simulink model "gm_parallel_phase_voltages_per_switching_state_6"  (R2022a)
settings: Solver=FixedStepDiscrete  StartTime=0.0  StopTime=10.0  RelTol=1e-3
undefined symbols (not defined in the file or in its folder): f_c, u_dc
libraries: hdlmdlgenlib x20
(part 1 of 5)
settings Model: Creator=Andre Merx  LastModifiedBy=Andre Merx
settings SolverCC: AlgebraicLoopSolver=TrustRegion
settings DataIOCC: LimitDataPoints=on  SaveOutput=off  SaveTime=off
settings OptimizationCC: BlockReduction=off  ConditionallyExecuteInputs=off  DefaultParameterBehavior=Inlined  LifeSpan=inf
settings DebuggingCC: AlgebraicLoopMsg=error  InheritedTsInSrcMsg=none  SingleTaskRateTransMsg=error  UnconnectedInputMsg=warning  UnconnectedOutputMsg=warning  UnconnectedLineMsg=warning  AllowSymbolicDim=off  StrictBusMsg=ErrorOnBusTreatedAsVector  SFUnexpectedBacktrackingDiag=warning  SFNoUnconditionalDefaultTransitionDiag=warning  SFExecutionAtInitializationDiag=none  SFMachineParentedDataDiag=warning  ArithmeticOperatorsInVariantConditions=warning
settings HardwareCC: ProdBitPerPointer=32  ProdBitPerSizeT=32  ProdBitPerPtrDiffT=32  ProdLargestAtomicFloat=None  ProdIntDivRoundTo=Undefined  ProdEndianess=Unspecified  ProdWordSize=32  ProdHWDeviceType=ASIC/FPGA->ASIC/FPGA  ProdEqTarget=off
settings SFSimCC: SimUseLocalCustomCode=off  CustomCodeUndefinedFunction=UseInterfaceOnly
settings RTWCC: RTWUseLocalCustomCode=off
settings CodeAppCC: StateflowObjectComments=on
settings GRTTargetCC: TargetLangStandard=C89/C90 (ANSI)
settings ConfigComp: CovScope=ReferencedModels  CovMetricSettings=dw  CovSaveCumulativeToWorkspaceVar=on  CovSaveSingleToWorkspaceVar=on  CovExternalEMLEnable=off  CovSFcnEnable=off

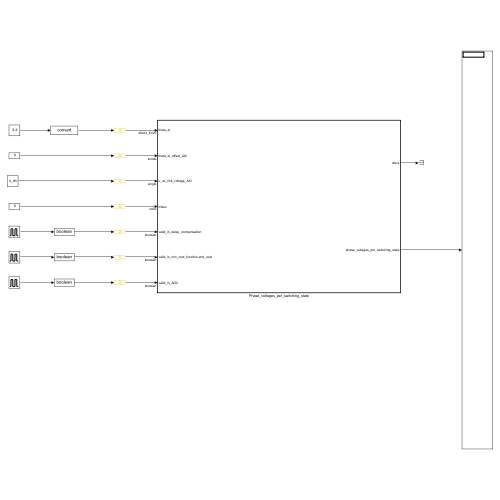
[thumbnail: Simulink's stored preview of the top-level diagram]
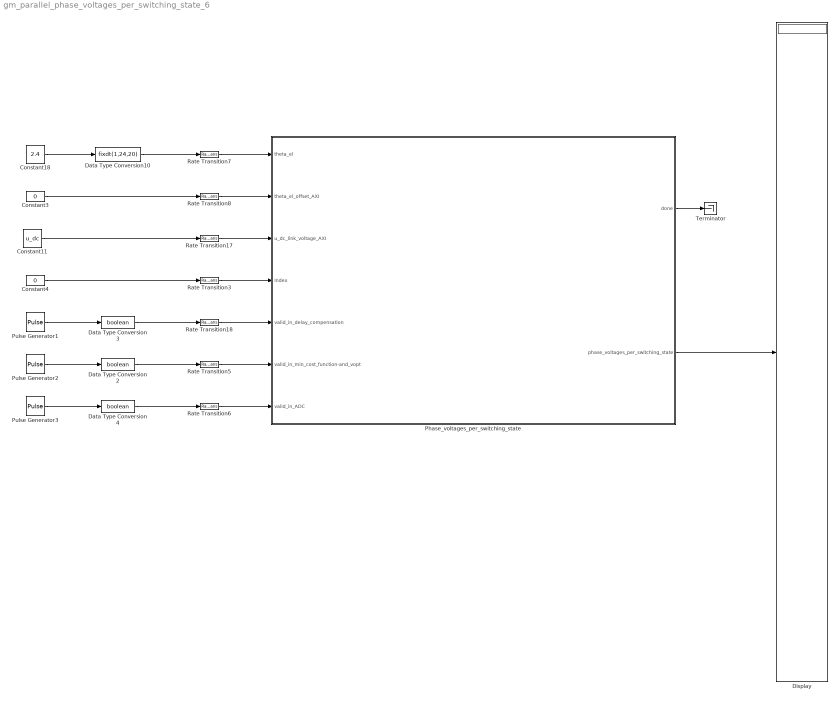
== system gm_parallel_phase_voltages_per_switching_state_6 ==
  Constant11 : Constant  Value=u_dc  OutDataTypeStr=single  SampleTime=-1
  Constant18 : Constant  Value=2.4
  Constant3 : Constant  Value=0  OutDataTypeStr=single  SampleTime=-1
  Constant4 : Constant  Value=0  OutDataTypeStr=int32  SampleTime=-1
  Data Type Conversion10 : DataTypeConversion  OutDataTypeStr=fixdt(1,24,20)  SaturateOnIntegerOverflow=off  RndMeth=Floor
  Data Type Conversion2 : DataTypeConversion  OutDataTypeStr=boolean  SaturateOnIntegerOverflow=off  RndMeth=Floor
  Data Type Conversion3 : DataTypeConversion  OutDataTypeStr=boolean  SaturateOnIntegerOverflow=off  RndMeth=Floor
  Data Type Conversion4 : DataTypeConversion  OutDataTypeStr=boolean  SaturateOnIntegerOverflow=off  RndMeth=Floor
  Display : Display
  Phase_voltages_per_switching_state : Subsystem  TreatAsAtomicUnit=on
  Pulse Generator1 : DiscretePulseGenerator  PulseType=Time based  Period=1/f_c
  Pulse Generator2 : DiscretePulseGenerator  PulseType=Time based  Period=1/f_c
  Pulse Generator3 : DiscretePulseGenerator  PulseType=Time based  Period=1/f_c
  Rate Transition{3,5..8,17..18} (7 alike) : RateTransition  OutPortSampleTime=Rt
  Terminator : Terminator
  wires:
  Phase_voltages_per_switching_state/2(phase_voltages_per_switching_state) -> Display/1
  Phase_voltages_per_switching_state/1(done) -> Terminator/1
  Data Type Conversion10/1 -> Rate Transition7/1
  Constant11/1 -> Rate Transition17/1
  Constant3/1 -> Rate Transition8/1
  Rate Transition17/1 -> Phase_voltages_per_switching_state/3(u_dc_link_voltage_AXI)
  Constant4/1 -> Rate Transition3/1
  Rate Transition7/1 -> Phase_voltages_per_switching_state/1(theta_el)
  Pulse Generator1/1 -> Data Type Conversion3/1
  Rate Transition8/1 -> Phase_voltages_per_switching_state/2(theta_el_offset_AXI)
  Constant18/1 -> Data Type Conversion10/1
  Rate Transition18/1 -> Phase_voltages_per_switching_state/5(valid_in_delay_compensation)
  Rate Transition3/1 -> Phase_voltages_per_switching_state/4(Index)
  Pulse Generator2/1 -> Data Type Conversion2/1
  Pulse Generator3/1 -> Data Type Conversion4/1
  Data Type Conversion4/1 -> Rate Transition6/1
  Rate Transition6/1 -> Phase_voltages_per_switching_state/7(valid_in_ADC)
  Rate Transition5/1 -> Phase_voltages_per_switching_state/6(valid_in_min_cost_function-and_vopt)
  Data Type Conversion3/1 -> Rate Transition18/1
  Data Type Conversion2/1 -> Rate Transition5/1

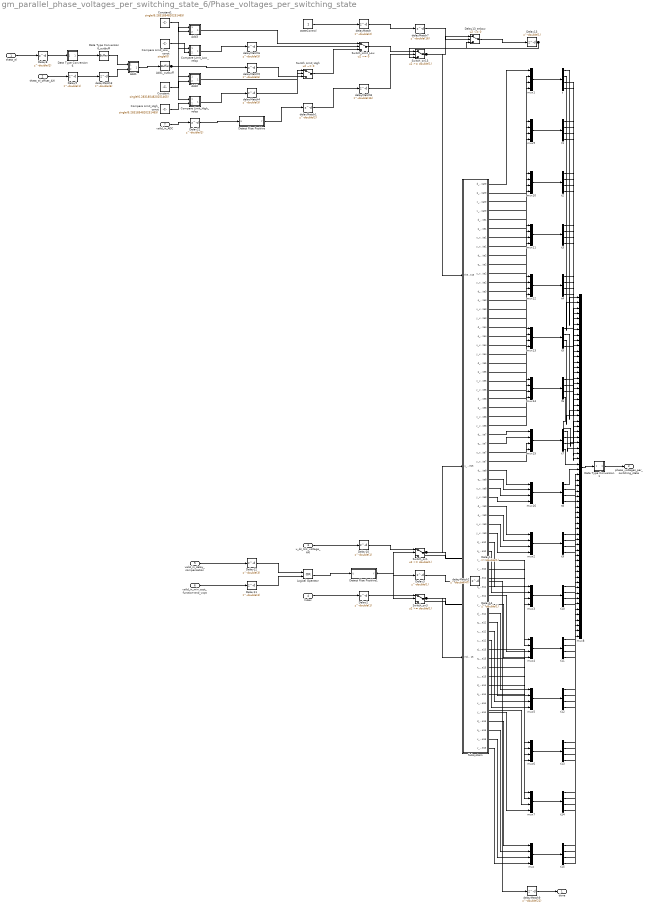
== system gm_parallel_phase_voltages_per_switching_state_6/Phase_voltages_per_switching_state ==
  theta_el : Inport  OutDataTypeStr=fixdt(1, 24, 20)  PortDimensions=1  SampleTime=1e-08
  theta_el_offset_AXI : Inport  Port=2  OutDataTypeStr=single  PortDimensions=1  SampleTime=1e-08
  u_dc_link_voltage_AXI : Inport  Port=3  OutDataTypeStr=single  PortDimensions=1  SampleTime=1e-08
  Index : Inport  Port=4  OutDataTypeStr=int32  PortDimensions=1  SampleTime=1e-08
  valid_in_delay_compensation : Inport  Port=5  OutDataTypeStr=boolean  PortDimensions=1  SampleTime=1e-08
  valid_in_min_cost_function-and_vopt : Inport  Port=6  OutDataTypeStr=boolean  PortDimensions=1  SampleTime=1e-08
  valid_in_ADC : Inport  Port=7  OutDataTypeStr=boolean  PortDimensions=1  SampleTime=1e-08
  Add1 : Subsystem
      mask Display: disp('NFP\nadd');
  Add1_outbuff : hdlmdlgenlib/Buffer
      settings: SourceProductBaseCode=SL
  Add2 : Subsystem
      mask Display: disp('NFP\nadd');
  Add3 : Subsystem
      mask Display: disp('NFP\nadd');
  Compare Limit_High_const : Constant  Value=single(6.2831854820251465)  OutDataTypeStr=single  SampleTime=1e-08
  Compare Limit_High_relop : Subsystem
      mask Display: disp('NFP\nrelop');
  Compare Limit_Low_const : Constant  Value=single(0)  OutDataTypeStr=single  SampleTime=1e-08
  Compare Limit_Low_relop : Subsystem
      mask Display: disp('NFP\nrelop');
  Constant : Constant  Value=single(6.2831854820251465)  OutDataTypeStr=single  SampleTime=1e-08
  Constant1 : Constant  Value=single(6.2831854820251465)  OutDataTypeStr=single  SampleTime=1e-08
  Data Type Conversion1 : Subsystem
      mask Display: disp('NFP\nconv');
  Data Type Conversion6 : Subsystem
      mask Display: disp('NFP\nconv');
  Data Type Conversion6_outbuff : hdlmdlgenlib/Buffer
      settings: SourceProductBaseCode=SL
  Delay{1..3,8..10,13..14,21} (9 alike) : Delay  DelayLength=double(1)  InitialCondition=0  SampleTime=1e-08
  Delay11 : Delay  DelayLength=double(3)  InitialCondition=0  SampleTime=1e-08
  Delay12 : Delay  DelayLength=double(3)  InitialCondition=0  SampleTime=1e-08
  Delay13_enbsw : Switch  Criteria=u2 ~= 0  Threshold=double(0)  OutDataTypeStr=single  SampleTime=1e-08  SaturateOnIntegerOverflow=off  InputSameDT=off
  Detect Rise Positive : Subsystem  mask(Detect Rise Positive){vinit=double(0), InputProcessing=Elements as channels (sample based), OutDataTypeStr=boolean}
      mask prompts: vinit "Simulink:masks:InitialCondition_MP"; InputProcessing "Simulink:masks:InputProcessing_MP"; OutDataTypeStr "Simulink:masks:OutputDataType_MP"
      mask help: Simulink:masks:DetectRisePositive_MD
      mask init:
      | InputProcessing = 'Elements as channels (sample based)';
      | OutDataTypeStr = 'boolean';
      | vinit = double(0);
      mask TypeOptions InputProcessing: Simulink:masks:ColumnsAsChannelsFrameBased | Simulink:masks:ElementsAsChannelsSampleBased
      mask TypeOptions OutDataTypeStr: Simulink:masks:uint8 | Simulink:masks:boolean
      mask Display: fprintf('U > 0\n&  NOT\nU/z > 0')
  Detect Rise Positive1 : Subsystem  mask(Detect Rise Positive){vinit=double(0), InputProcessing=Elements as channels (sample based), OutDataTypeStr=boolean}
      mask prompts: vinit "Simulink:masks:InitialCondition_MP"; InputProcessing "Simulink:masks:InputProcessing_MP"; OutDataTypeStr "Simulink:masks:OutputDataType_MP"
      mask help: Simulink:masks:DetectRisePositive_MD
      mask init:
      | InputProcessing = 'Elements as channels (sample based)';
      | OutDataTypeStr = 'boolean';
      | vinit = double(0);
      mask TypeOptions InputProcessing: Simulink:masks:ColumnsAsChannelsFrameBased | Simulink:masks:ElementsAsChannelsSampleBased
      mask TypeOptions OutDataTypeStr: Simulink:masks:uint8 | Simulink:masks:boolean
      mask Display: fprintf('U > 0\n&  NOT\nU/z > 0')
  Logical Operator : Logic  Operator=OR  AllPortsSameDT=off  OutDataTypeStr=boolean  SampleTime=1e-08
  Subsystem : Subsystem
  Switch_Limit_High : Switch  Criteria=u2 ~= 0  Threshold=double(0)  OutDataTypeStr=single  SampleTime=1e-08  SaturateOnIntegerOverflow=off  InputSameDT=off
  Switch_Limit_Low : Switch  Criteria=u2 ~= 0  Threshold=double(0)  OutDataTypeStr=single  SampleTime=1e-08  SaturateOnIntegerOverflow=off  InputSameDT=off
  Switch_on1 : Switch  Threshold=double(1)  OutDataTypeStr=single  RndMeth=Simplest  SampleTime=1e-08  SaturateOnIntegerOverflow=off  InputSameDT=off
  Switch_on13 : Switch  Threshold=double(1)  OutDataTypeStr=single  RndMeth=Simplest  SampleTime=1e-08  SaturateOnIntegerOverflow=off  InputSameDT=off
  Switch_on3 : Switch  Threshold=double(1)  OutDataTypeStr=int32  RndMeth=Simplest  SampleTime=1e-08  SaturateOnIntegerOverflow=off  InputSameDT=off
  delayMatch : Delay  DelayLength=double(2)  InitialCondition=0  SampleTime=1e-08
  delayMatch1 : Delay  DelayLength=double(2)  InitialCondition=0  SampleTime=1e-08
  delayMatch2 : Delay  DelayLength=double(47)  InitialCondition=0  SampleTime=1e-08
  delayMatch3 : Delay  DelayLength=double(6)  InitialCondition=0  SampleTime=1e-08
  delayMatch4 : Delay  DelayLength=double(5)  InitialCondition=0  SampleTime=1e-08
  delayMatch5 : Delay  DelayLength=double(6)  InitialCondition=0  SampleTime=1e-08
  delayMatch6 : Delay  DelayLength=double(5)  InitialCondition=0  SampleTime=1e-08
  delayMatch7 : Delay  DelayLength=double(16)  InitialCondition=0  SampleTime=1e-08
  delayMatch8 : Delay  DelayLength=double(16)  InitialCondition=0  SampleTime=1e-08
  delayMatch9 : Delay  DelayLength=double(21)  InitialCondition=0  SampleTime=1e-08
  mux{,1..7,9..16} (16 alike) : Mux
  mux8 : Mux  Inputs=64
  stateControl : Constant  OutDataTypeStr=boolean  SampleTime=1e-08
  t{,1..15} (16 alike) : Demux
  done : Outport  SampleTime=1e-08
  phase_voltages_per_switching_state : Outport  Port=2  SampleTime=1e-08
  wires:
  theta_el/1 -> Delay8/1
  theta_el_offset_AXI/1 -> Delay9/1
  u_dc_link_voltage_AXI/1 -> Delay10/1
  Index/1 -> Delay2/1
  valid_in_delay_compensation/1 -> Delay12/1
  valid_in_min_cost_function-and_vopt/1 -> Delay11/1
  valid_in_ADC/1 -> Delay21/1
  delayMatch5/1 -> Switch_Limit_High/3
  Constant/1 -> Add2/2(In2)
  Constant1/1 -> Add3/2(In2)
  Data Type Conversion6_outbuff/1 -> Add1/1(In1)
  Delay10/1 -> Switch_on1/1
  Delay11/1 -> Logical Operator/2
  Delay12/1 -> Logical Operator/1
  Delay2/1 -> Switch_on3/1
  Delay21/1 -> Detect Rise Positive/1(U)
  delayMatch9/1 -> done/1
  Delay8/1 -> Data Type Conversion6/1(In1)
  delayMatch3/1 -> Add1/2(In2)
  delayMatch8/1 -> Switch_on13/2
  Detect Rise Positive1/1(Y) -> Delay3/1, Switch_on1/2, Switch_on3/2
  Logical Operator/1 -> Detect Rise Positive1/1(U)
  mux/1 -> t15/1
  mux1/1 -> t/1
  mux2/1 -> t9/1
  mux3/1 -> t10/1
  mux4/1 -> t11/1
  mux5/1 -> t12/1
  mux6/1 -> t13/1
  mux7/1 -> t14/1
  mux8/1 -> Data Type Conversion1/1(In1)
  mux9/1 -> t1/1
  mux10/1 -> t2/1
  mux11/1 -> t3/1
  mux12/1 -> t4/1
  mux13/1 -> t5/1
  mux14/1 -> t6/1
  mux15/1 -> t7/1
  mux16/1 -> t8/1
  Subsystem/1(d_voltage_per_switching_state) -> mux1/1
  Subsystem/2(q_voltage_per_switching_state) -> mux1/2
  Subsystem/3(x_voltage_per_switching_state) -> mux1/3
  Subsystem/4(y_voltage_per_switching_state) -> mux1/4
  Subsystem/5(d_voltage_per_switching_state1) -> mux9/1
  Subsystem/6(q_voltage_per_switching_state1) -> mux9/2
  Subsystem/7(x_voltage_per_switching_state1) -> mux9/3
  Subsystem/8(y_voltage_per_switching_state1) -> mux9/4
  Subsystem/9(d_voltage_per_switching_state2) -> mux10/1
  Subsystem/10(q_voltage_per_switching_state2) -> mux10/2
  Subsystem/11(x_voltage_per_switching_state2) -> mux10/3
  Subsystem/12(y_voltage_per_switching_state2) -> mux10/4
  Subsystem/13(d_voltage_per_switching_state3) -> mux11/1
  Subsystem/14(q_voltage_per_switching_state3) -> mux11/2
  Subsystem/15(x_voltage_per_switching_state3) -> mux11/3
  Subsystem/16(y_voltage_per_switching_state3) -> mux11/4
  Subsystem/17(d_voltage_per_switching_state4) -> mux12/1
  Subsystem/18(q_voltage_per_switching_state4) -> mux12/2
  Subsystem/19(x_voltage_per_switching_state4) -> mux12/3
  Subsystem/20(y_voltage_per_switching_state4) -> mux12/4
  Subsystem/21(d_voltage_per_switching_state5) -> mux13/1
  Subsystem/22(q_voltage_per_switching_state5) -> mux13/2
  Subsystem/23(x_voltage_per_switching_state5) -> mux13/3
  Subsystem/24(y_voltage_per_switching_state5) -> mux13/4
  Subsystem/25(d_voltage_per_switching_state6) -> mux14/1
  Subsystem/26(q_voltage_per_switching_state6) -> mux14/2
  Subsystem/27(x_voltage_per_switching_state6) -> mux14/3
  Subsystem/28(y_voltage_per_switching_state6) -> mux14/4
  Subsystem/29(d_voltage_per_switching_state7) -> mux15/1
  Subsystem/30(q_voltage_per_switching_state7) -> mux15/2
  Subsystem/31(x_voltage_per_switching_state7) -> mux15/3
  Subsystem/32(y_voltage_per_switching_state7) -> mux15/4
  Subsystem/33(d_voltage_per_switching_state8) -> mux16/1
  Subsystem/34(q_voltage_per_switching_state8) -> mux16/2
  Subsystem/35(x_voltage_per_switching_state8) -> mux16/3
  Subsystem/36(y_voltage_per_switching_state8) -> mux16/4
  Subsystem/37(d_voltage_per_switching_state9) -> mux2/1
  Subsystem/38(q_voltage_per_switching_state9) -> mux2/2
  Subsystem/39(x_voltage_per_switching_state9) -> mux2/3
  Subsystem/40(y_voltage_per_switching_state9) -> mux2/4
  Subsystem/41(d_voltage_per_switching_state10) -> mux3/1
  Subsystem/42(q_voltage_per_switching_state10) -> mux3/2
  Subsystem/43(x_voltage_per_switching_state10) -> mux3/3
  Subsystem/44(y_voltage_per_switching_state10) -> mux3/4
  Subsystem/45(d_voltage_per_switching_state11) -> mux4/1
  Subsystem/46(q_voltage_per_switching_state11) -> mux4/2
  Subsystem/47(x_voltage_per_switching_state11) -> mux4/3
  Subsystem/48(y_voltage_per_switching_state11) -> mux4/4
  Subsystem/49(d_voltage_per_switching_state12) -> mux5/1
  Subsystem/50(q_voltage_per_switching_state12) -> mux5/2
  Subsystem/51(x_voltage_per_switching_state12) -> mux5/3
  Subsystem/52(y_voltage_per_switching_state12) -> mux5/4
  Subsystem/53(d_voltage_per_switching_state13) -> mux6/1
  Subsystem/54(q_voltage_per_switching_state13) -> mux6/2
  Subsystem/55(x_voltage_per_switching_state13) -> mux6/3
  Subsystem/56(y_voltage_per_switching_state13) -> mux6/4
  Subsystem/57(d_voltage_per_switching_state14) -> mux7/1
  Subsystem/58(q_voltage_per_switching_state14) -> mux7/2
  Subsystem/59(x_voltage_per_switching_state14) -> mux7/3
  Subsystem/60(y_voltage_per_switching_state14) -> mux7/4
  Subsystem/61(d_voltage_per_switching_state15) -> mux/1
  Subsystem/62(q_voltage_per_switching_state15) -> mux/2
  Subsystem/63(x_voltage_per_switching_state15) -> mux/3
  Subsystem/64(y_voltage_per_switching_state15) -> mux/4
  Switch_Limit_High/1 -> Switch_Limit_Low/3
  Switch_Limit_Low/1 -> Switch_on13/1
  Switch_on1/1 -> Subsystem/2(u_dc_link_voltage15), Delay1/1
  Switch_on3/1 -> Subsystem/3(Index 15), Delay14/1
  Add1_outbuff/1 -> Compare Limit_Low_relop/1(In1), Compare Limit_High_relop/1(In1), Add3/1(In1), Add2/1(In1), delayMatch5/1
  delayMatch4/1 -> Switch_Limit_High/2
  delayMatch6/1 -> Switch_Limit_Low/2
  Compare Limit_High_const/1 -> Compare Limit_High_relop/2(In2)
  Compare Limit_Low_const/1 -> Compare Limit_Low_relop/2(In2)
  t/1 -> mux8/1
  t/2 -> mux8/2
  t/3 -> mux8/3
  t/4 -> mux8/4
  t1/1 -> mux8/5
  t1/2 -> mux8/6
  t1/3 -> mux8/7
  t1/4 -> mux8/8
  t2/1 -> mux8/9
  t2/2 -> mux8/10
  t2/3 -> mux8/11
  t2/4 -> mux8/12
  t3/1 -> mux8/13
  t3/2 -> mux8/14
  t3/3 -> mux8/15
  t3/4 -> mux8/16
  t4/1 -> mux8/17
  t4/2 -> mux8/18
  t4/3 -> mux8/19
  t4/4 -> mux8/20
  t5/1 -> mux8/21
  t5/2 -> mux8/22
  t5/3 -> mux8/23
  t5/4 -> mux8/24
  t6/1 -> mux8/25
  t6/2 -> mux8/26
  t6/3 -> mux8/27
  t6/4 -> mux8/28
  t7/1 -> mux8/29
  t7/2 -> mux8/30
  t7/3 -> mux8/31
  t7/4 -> mux8/32
  t8/1 -> mux8/33
  t8/2 -> mux8/34
  t8/3 -> mux8/35
  t8/4 -> mux8/36
  t9/1 -> mux8/37
  t9/2 -> mux8/38
  t9/3 -> mux8/39
  t9/4 -> mux8/40
  t10/1 -> mux8/41
  t10/2 -> mux8/42
  t10/3 -> mux8/43
  t10/4 -> mux8/44
  t11/1 -> mux8/45
  t11/2 -> mux8/46
  t11/3 -> mux8/47
  t11/4 -> mux8/48
  t12/1 -> mux8/49
  t12/2 -> mux8/50
  t12/3 -> mux8/51
  t12/4 -> mux8/52
  t13/1 -> mux8/53
  t13/2 -> mux8/54
  t13/3 -> mux8/55
  t13/4 -> mux8/56
  t14/1 -> mux8/57
  t14/2 -> mux8/58
  t14/3 -> mux8/59
  t14/4 -> mux8/60
  t15/1 -> mux8/61
  t15/2 -> mux8/62
  t15/3 -> mux8/63
  t15/4 -> mux8/64
  delayMatch7/1 -> Delay13_enbsw/2
  stateControl/1 -> delayMatch/1
  Detect Rise Positive/1(Y) -> delayMatch1/1
  Delay3/1 -> delayMatch2/1
  Add1/1(Out1) -> Add1_outbuff/1
  Add2/1(Out1) -> Switch_Limit_High/1
  Add3/1(Out1) -> Switch_Limit_Low/1
  Compare Limit_High_relop/1(Out1) -> delayMatch4/1
  Compare Limit_Low_relop/1(Out1) -> delayMatch6/1
  Data Type Conversion1/1(Out1) -> phase_voltages_per_switching_state/1
  Data Type Conversion6/1(Out1) -> Data Type Conversion6_outbuff/1
  Delay9/1 -> delayMatch3/1
  delayMatch/1 -> delayMatch7/1
  delayMatch1/1 -> delayMatch8/1
  delayMatch2/1 -> delayMatch9/1
  Switch_on13/1 -> Subsystem/1(theta_el_with_offset15), Delay13_enbsw/1
  Delay13_enbsw/1 -> Delay13/1
  Delay13/1 -> Switch_on13/3, Delay13_enbsw/3
  Delay1/1 -> Switch_on1/3
  Delay14/1 -> Switch_on3/3

== system gm_parallel_phase_voltages_per_switching_state_6/Phase_voltages_per_switching_state/Add1 ==
  In1 : Inport
  In2 : Inport  Port=2
  Add1 : Sum  Inputs=+-  OutDataTypeStr=single  SampleTime=1e-08
  Add1_pd1 : Delay  DelayLength=6
  Out1 : Outport
  wires:
  In1/1 -> Add1/1
  In2/1 -> Add1/2
  Add1/1 -> Add1_pd1/1
  Add1_pd1/1 -> Out1/1

== system gm_parallel_phase_voltages_per_switching_state_6/Phase_voltages_per_switching_state/Add2 ==
  In1 : Inport
  In2 : Inport  Port=2
  Add2 : Sum  Inputs=+-  OutDataTypeStr=single  SampleTime=1e-08
  Add2_pd1 : Delay  DelayLength=6
  Out1 : Outport
  wires:
  In1/1 -> Add2/1
  In2/1 -> Add2/2
  Add2/1 -> Add2_pd1/1
  Add2_pd1/1 -> Out1/1

== system gm_parallel_phase_voltages_per_switching_state_6/Phase_voltages_per_switching_state/Add3 ==
  In1 : Inport
  In2 : Inport  Port=2
  Add3 : Sum  OutDataTypeStr=single  SampleTime=1e-08
  Add3_pd1 : Delay  DelayLength=6
  Out1 : Outport
  wires:
  In1/1 -> Add3/1
  In2/1 -> Add3/2
  Add3/1 -> Add3_pd1/1
  Add3_pd1/1 -> Out1/1

== system gm_parallel_phase_voltages_per_switching_state_6/Phase_voltages_per_switching_state/Compare Limit_High_relop ==
  In1 : Inport
  In2 : Inport  Port=2
  Compare Limit_High_relop : RelationalOperator  OutDataTypeStr=boolean  SampleTime=1e-08
  Compare Limit_High_relop_pd1 : Delay  DelayLength=1
  Out1 : Outport
  wires:
  In1/1 -> Compare Limit_High_relop/1
  In2/1 -> Compare Limit_High_relop/2
  Compare Limit_High_relop/1 -> Compare Limit_High_relop_pd1/1
  Compare Limit_High_relop_pd1/1 -> Out1/1

== system gm_parallel_phase_voltages_per_switching_state_6/Phase_voltages_per_switching_state/Compare Limit_Low_relop ==
  In1 : Inport
  In2 : Inport  Port=2
  Compare Limit_Low_relop : RelationalOperator  Operator=<  OutDataTypeStr=boolean  SampleTime=1e-08
  Compare Limit_Low_relop_pd1 : Delay  DelayLength=1
  Out1 : Outport
  wires:
  In1/1 -> Compare Limit_Low_relop/1
  In2/1 -> Compare Limit_Low_relop/2
  Compare Limit_Low_relop/1 -> Compare Limit_Low_relop_pd1/1
  Compare Limit_Low_relop_pd1/1 -> Out1/1

== system gm_parallel_phase_voltages_per_switching_state_6/Phase_voltages_per_switching_state/Data Type Conversion1 ==
  In1 : Inport
  Data Type Conversion1 : DataTypeConversion  OutDataTypeStr=fixdt(1, 24, 11)  SampleTime=1e-08  SaturateOnIntegerOverflow=off  RndMeth=Floor
  Data Type Conversion1_pd1 : Delay  DelayLength=6
  Out1 : Outport
  wires:
  In1/1 -> Data Type Conversion1/1
  Data Type Conversion1/1 -> Data Type Conversion1_pd1/1
  Data Type Conversion1_pd1/1 -> Out1/1

== system gm_parallel_phase_voltages_per_switching_state_6/Phase_voltages_per_switching_state/Data Type Conversion6 ==
  In1 : Inport
  Data Type Conversion6 : DataTypeConversion  OutDataTypeStr=single  RndMeth=Nearest  SampleTime=1e-08  SaturateOnIntegerOverflow=off
  Data Type Conversion6_pd1 : Delay  DelayLength=6
  Out1 : Outport
  wires:
  In1/1 -> Data Type Conversion6/1
  Data Type Conversion6/1 -> Data Type Conversion6_pd1/1
  Data Type Conversion6_pd1/1 -> Out1/1

== system gm_parallel_phase_voltages_per_switching_state_6/Phase_voltages_per_switching_state/Detect Rise Positive ==
  note: Edge
  note: U(k)
  U : Inport  OutDataTypeStr=boolean  SampleTime=1e-08
  Delay Input1 : UnitDelay  Description=Store in Global RAM  DisableCoverage=on  InitialCondition=vinit  SampleTime=-1  HasFrameUpgradeWarning=on
  FixPt Relational Operator : RelationalOperator  Operator=>  OutDataTypeStr=boolean  ZeroCross=off  InputSameDT=off
  Positive : Subsystem  mask(Compare To Zero){relop=>, OutDataTypeStr=boolean, ZeroCross=off}
      mask prompts: relop "Simulink:masks:Operator_MP"; OutDataTypeStr "Simulink:masks:OutputDataType_MP"; ZeroCross "Simulink:masks:EnableZerocrossingDetection_MP"
      mask help: Simulink:masks:CompareToZero_MD
      mask init:
      | OutDataTypeStr = 'boolean';
      | ZeroCross = 'off';
      | blkName = 'parallel_phase_voltages_per_switching_state_6/Phase_voltages_per_switching_state/Detect Rise\nPositive/Positive';
      | relop = '>';
      | setValue = 'boolean';
      mask TypeOptions relop: == | ~= | < | <= | >= | >
      mask TypeOptions OutDataTypeStr: Simulink:masks:uint8 | Simulink:masks:boolean
      mask Callback ZeroCross: sl('zeroCrossEnable', gcbh);
      mask Display: disp([relop,' 0'])
  Y : Outport  SampleTime=1e-08
  wires:
  Delay Input1/1 -> FixPt Relational Operator/2
  FixPt Relational Operator/1 -> Y/1
  Positive/1(y) -> FixPt Relational Operator/1, Delay Input1/1
  U/1 -> Positive/1(u)

== system gm_parallel_phase_voltages_per_switching_state_6/Phase_voltages_per_switching_state/Detect Rise Positive1 ==
  note: Edge
  note: U(k)
  U : Inport  OutDataTypeStr=boolean  SampleTime=1e-08
  Delay Input1 : UnitDelay  Description=Store in Global RAM  DisableCoverage=on  InitialCondition=vinit  SampleTime=-1  HasFrameUpgradeWarning=on
  FixPt Relational Operator : RelationalOperator  Operator=>  OutDataTypeStr=boolean  ZeroCross=off  InputSameDT=off
  Positive : Subsystem  mask(Compare To Zero){relop=>, OutDataTypeStr=boolean, ZeroCross=off}
      mask prompts: relop "Simulink:masks:Operator_MP"; OutDataTypeStr "Simulink:masks:OutputDataType_MP"; ZeroCross "Simulink:masks:EnableZerocrossingDetection_MP"
      mask help: Simulink:masks:CompareToZero_MD
      mask init:
      | OutDataTypeStr = 'boolean';
      | ZeroCross = 'off';
      | blkName = 'parallel_phase_voltages_per_switching_state_6/Phase_voltages_per_switching_state/Detect Rise\nPositive1/Positive';
      | relop = '>';
      | setValue = 'boolean';
      mask TypeOptions relop: == | ~= | < | <= | >= | >
      mask TypeOptions OutDataTypeStr: Simulink:masks:uint8 | Simulink:masks:boolean
      mask Callback ZeroCross: sl('zeroCrossEnable', gcbh);
      mask Display: disp([relop,' 0'])
  Y : Outport  SampleTime=1e-08
  wires:
  Delay Input1/1 -> FixPt Relational Operator/2
  FixPt Relational Operator/1 -> Y/1
  Positive/1(y) -> FixPt Relational Operator/1, Delay Input1/1
  U/1 -> Positive/1(u)

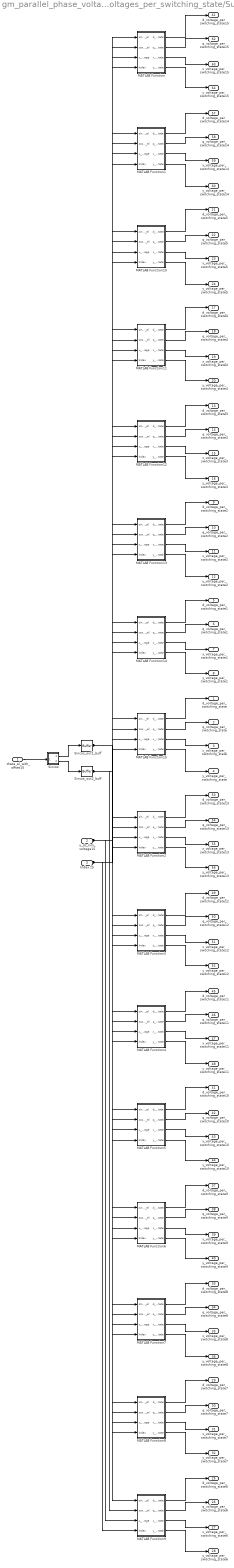
== system gm_parallel_phase_voltages_per_switching_state_6/Phase_voltages_per_switching_state/Subsystem ==
  theta_el_with_offset15 : Inport  OutDataTypeStr=single  PortDimensions=1  SampleTime=1e-08
  u_dc_link_voltage15 : Inport  Port=2  OutDataTypeStr=single  PortDimensions=1  SampleTime=1e-08
  Index 15 : Inport  Port=3  OutDataTypeStr=int32  PortDimensions=1  SampleTime=1e-08
  MATLAB Function : Subsystem
  MATLAB Function1 : Subsystem
  MATLAB Function10 : Subsystem
  MATLAB Function11 : Subsystem
  MATLAB Function12 : Subsystem
  MATLAB Function13 : Subsystem
  MATLAB Function14 : Subsystem
  MATLAB Function15 : Subsystem
  MATLAB Function2 : Subsystem
  MATLAB Function3 : Subsystem
  MATLAB Function4 : Subsystem
  MATLAB Function5 : Subsystem
  MATLAB Function6 : Subsystem
  MATLAB Function7 : Subsystem
  MATLAB Function8 : Subsystem
  MATLAB Function9 : Subsystem
  Sincos : Subsystem
      mask Display: disp('NFP\ntrig2');
  Sincos_out1_buff : hdlmdlgenlib/Buffer
      settings: SourceProductBaseCode=SL
  Sincos_out2_buff : hdlmdlgenlib/Buffer
      settings: SourceProductBaseCode=SL
  d_voltage_per_switching_state : Outport  SampleTime=1e-08
  q_voltage_per_switching_state : Outport  Port=2  SampleTime=1e-08
  x_voltage_per_switching_state : Outport  Port=3  SampleTime=1e-08
  y_voltage_per_switching_state : Outport  Port=4  SampleTime=1e-08
  d_voltage_per_switching_state1 : Outport  Port=5  SampleTime=1e-08
  q_voltage_per_switching_state1 : Outport  Port=6  SampleTime=1e-08
  x_voltage_per_switching_state1 : Outport  Port=7  SampleTime=1e-08
  y_voltage_per_switching_state1 : Outport  Port=8  SampleTime=1e-08
  d_voltage_per_switching_state2 : Outport  Port=9  SampleTime=1e-08
  q_voltage_per_switching_state2 : Outport  Port=10  SampleTime=1e-08
  x_voltage_per_switching_state2 : Outport  Port=11  SampleTime=1e-08
  y_voltage_per_switching_state2 : Outport  Port=12  SampleTime=1e-08
  d_voltage_per_switching_state3 : Outport  Port=13  SampleTime=1e-08
  q_voltage_per_switching_state3 : Outport  Port=14  SampleTime=1e-08
  x_voltage_per_switching_state3 : Outport  Port=15  SampleTime=1e-08
  y_voltage_per_switching_state3 : Outport  Port=16  SampleTime=1e-08
  d_voltage_per_switching_state4 : Outport  Port=17  SampleTime=1e-08
  q_voltage_per_switching_state4 : Outport  Port=18  SampleTime=1e-08
  x_voltage_per_switching_state4 : Outport  Port=19  SampleTime=1e-08
  y_voltage_per_switching_state4 : Outport  Port=20  SampleTime=1e-08
  d_voltage_per_switching_state5 : Outport  Port=21  SampleTime=1e-08
  q_voltage_per_switching_state5 : Outport  Port=22  SampleTime=1e-08
  x_voltage_per_switching_state5 : Outport  Port=23  SampleTime=1e-08
  y_voltage_per_switching_state5 : Outport  Port=24  SampleTime=1e-08
  d_voltage_per_switching_state6 : Outport  Port=25  SampleTime=1e-08
  q_voltage_per_switching_state6 : Outport  Port=26  SampleTime=1e-08
  x_voltage_per_switching_state6 : Outport  Port=27  SampleTime=1e-08
  y_voltage_per_switching_state6 : Outport  Port=28  SampleTime=1e-08
  d_voltage_per_switching_state7 : Outport  Port=29  SampleTime=1e-08
  q_voltage_per_switching_state7 : Outport  Port=30  SampleTime=1e-08
  x_voltage_per_switching_state7 : Outport  Port=31  SampleTime=1e-08
  y_voltage_per_switching_state7 : Outport  Port=32  SampleTime=1e-08
  d_voltage_per_switching_state8 : Outport  Port=33  SampleTime=1e-08
  q_voltage_per_switching_state8 : Outport  Port=34  SampleTime=1e-08
  x_voltage_per_switching_state8 : Outport  Port=35  SampleTime=1e-08
  y_voltage_per_switching_state8 : Outport  Port=36  SampleTime=1e-08
  d_voltage_per_switching_state9 : Outport  Port=37  SampleTime=1e-08
  q_voltage_per_switching_state9 : Outport  Port=38  SampleTime=1e-08
  x_voltage_per_switching_state9 : Outport  Port=39  SampleTime=1e-08
  y_voltage_per_switching_state9 : Outport  Port=40  SampleTime=1e-08
  d_voltage_per_switching_state10 : Outport  Port=41  SampleTime=1e-08
  q_voltage_per_switching_state10 : Outport  Port=42  SampleTime=1e-08
  x_voltage_per_switching_state10 : Outport  Port=43  SampleTime=1e-08
  y_voltage_per_switching_state10 : Outport  Port=44  SampleTime=1e-08
  d_voltage_per_switching_state11 : Outport  Port=45  SampleTime=1e-08
  q_voltage_per_switching_state11 : Outport  Port=46  SampleTime=1e-08
  x_voltage_per_switching_state11 : Outport  Port=47  SampleTime=1e-08
  y_voltage_per_switching_state11 : Outport  Port=48  SampleTime=1e-08
  d_voltage_per_switching_state12 : Outport  Port=49  SampleTime=1e-08
  q_voltage_per_switching_state12 : Outport  Port=50  SampleTime=1e-08
  x_voltage_per_switching_state12 : Outport  Port=51  SampleTime=1e-08
  y_voltage_per_switching_state12 : Outport  Port=52  SampleTime=1e-08
  d_voltage_per_switching_state13 : Outport  Port=53  SampleTime=1e-08
  q_voltage_per_switching_state13 : Outport  Port=54  SampleTime=1e-08
  x_voltage_per_switching_state13 : Outport  Port=55  SampleTime=1e-08
  y_voltage_per_switching_state13 : Outport  Port=56  SampleTime=1e-08
  d_voltage_per_switching_state14 : Outport  Port=57  SampleTime=1e-08
  q_voltage_per_switching_state14 : Outport  Port=58  SampleTime=1e-08
  x_voltage_per_switching_state14 : Outport  Port=59  SampleTime=1e-08
  y_voltage_per_switching_state14 : Outport  Port=60  SampleTime=1e-08
  d_voltage_per_switching_state15 : Outport  Port=61  SampleTime=1e-08
  q_voltage_per_switching_state15 : Outport  Port=62  SampleTime=1e-08
  x_voltage_per_switching_state15 : Outport  Port=63  SampleTime=1e-08
  y_voltage_per_switching_state15 : Outport  Port=64  SampleTime=1e-08
  wires:
  MATLAB Function/1(d_voltage_per_switching_state) -> d_voltage_per_switching_state15/1
  MATLAB Function/2(q_voltage_per_switching_state) -> q_voltage_per_switching_state15/1
  MATLAB Function/3(x_voltage_per_switching_state) -> x_voltage_per_switching_state15/1
  MATLAB Function/4(y_voltage_per_switching_state) -> y_voltage_per_switching_state15/1
  MATLAB Function1/1(d_voltage_per_switching_state) -> d_voltage_per_switching_state14/1
  MATLAB Function1/2(q_voltage_per_switching_state) -> q_voltage_per_switching_state14/1
  MATLAB Function1/3(x_voltage_per_switching_state) -> x_voltage_per_switching_state14/1
  MATLAB Function1/4(y_voltage_per_switching_state) -> y_voltage_per_switching_state14/1
  MATLAB Function10/1(d_voltage_per_switching_state) -> d_voltage_per_switching_state5/1
  MATLAB Function10/2(q_voltage_per_switching_state) -> q_voltage_per_switching_state5/1
  MATLAB Function10/3(x_voltage_per_switching_state) -> x_voltage_per_switching_state5/1
  MATLAB Function10/4(y_voltage_per_switching_state) -> y_voltage_per_switching_state5/1
  MATLAB Function11/1(d_voltage_per_switching_state) -> d_voltage_per_switching_state4/1
  MATLAB Function11/2(q_voltage_per_switching_state) -> q_voltage_per_switching_state4/1
  MATLAB Function11/3(x_voltage_per_switching_state) -> x_voltage_per_switching_state4/1
  MATLAB Function11/4(y_voltage_per_switching_state) -> y_voltage_per_switching_state4/1
  MATLAB Function12/1(d_voltage_per_switching_state) -> d_voltage_per_switching_state3/1
  MATLAB Function12/2(q_voltage_per_switching_state) -> q_voltage_per_switching_state3/1
  MATLAB Function12/3(x_voltage_per_switching_state) -> x_voltage_per_switching_state3/1
  MATLAB Function12/4(y_voltage_per_switching_state) -> y_voltage_per_switching_state3/1
  MATLAB Function13/1(d_voltage_per_switching_state) -> d_voltage_per_switching_state2/1
  MATLAB Function13/2(q_voltage_per_switching_state) -> q_voltage_per_switching_state2/1
  MATLAB Function13/3(x_voltage_per_switching_state) -> x_voltage_per_switching_state2/1
  MATLAB Function13/4(y_voltage_per_switching_state) -> y_voltage_per_switching_state2/1
  MATLAB Function14/1(d_voltage_per_switching_state) -> d_voltage_per_switching_state1/1
  MATLAB Function14/2(q_voltage_per_switching_state) -> q_voltage_per_switching_state1/1
  MATLAB Function14/3(x_voltage_per_switching_state) -> x_voltage_per_switching_state1/1
  MATLAB Function14/4(y_voltage_per_switching_state) -> y_voltage_per_switching_state1/1
  MATLAB Function15/1(d_voltage_per_switching_state) -> d_voltage_per_switching_state/1
  MATLAB Function15/2(q_voltage_per_switching_state) -> q_voltage_per_switching_state/1
  MATLAB Function15/3(x_voltage_per_switching_state) -> x_voltage_per_switching_state/1
  MATLAB Function15/4(y_voltage_per_switching_state) -> y_voltage_per_switching_state/1
  MATLAB Function2/1(d_voltage_per_switching_state) -> d_voltage_per_switching_state13/1
  MATLAB Function2/2(q_voltage_per_switching_state) -> q_voltage_per_switching_state13/1
  MATLAB Function2/3(x_voltage_per_switching_state) -> x_voltage_per_switching_state13/1
  MATLAB Function2/4(y_voltage_per_switching_state) -> y_voltage_per_switching_state13/1
  MATLAB Function3/1(d_voltage_per_switching_state) -> d_voltage_per_switching_state12/1
  MATLAB Function3/2(q_voltage_per_switching_state) -> q_voltage_per_switching_state12/1
  MATLAB Function3/3(x_voltage_per_switching_state) -> x_voltage_per_switching_state12/1
  MATLAB Function3/4(y_voltage_per_switching_state) -> y_voltage_per_switching_state12/1
  MATLAB Function4/1(d_voltage_per_switching_state) -> d_voltage_per_switching_state11/1
  MATLAB Function4/2(q_voltage_per_switching_state) -> q_voltage_per_switching_state11/1
  MATLAB Function4/3(x_voltage_per_switching_state) -> x_voltage_per_switching_state11/1
  MATLAB Function4/4(y_voltage_per_switching_state) -> y_voltage_per_switching_state11/1
  MATLAB Function5/1(d_voltage_per_switching_state) -> d_voltage_per_switching_state10/1
  MATLAB Function5/2(q_voltage_per_switching_state) -> q_voltage_per_switching_state10/1
  MATLAB Function5/3(x_voltage_per_switching_state) -> x_voltage_per_switching_state10/1
  MATLAB Function5/4(y_voltage_per_switching_state) -> y_voltage_per_switching_state10/1
  MATLAB Function6/1(d_voltage_per_switching_state) -> d_voltage_per_switching_state9/1
  MATLAB Function6/2(q_voltage_per_switching_state) -> q_voltage_per_switching_state9/1
  MATLAB Function6/3(x_voltage_per_switching_state) -> x_voltage_per_switching_state9/1
  MATLAB Function6/4(y_voltage_per_switching_state) -> y_voltage_per_switching_state9/1
  MATLAB Function7/1(d_voltage_per_switching_state) -> d_voltage_per_switching_state8/1
  MATLAB Function7/2(q_voltage_per_switching_state) -> q_voltage_per_switching_state8/1
  MATLAB Function7/3(x_voltage_per_switching_state) -> x_voltage_per_switching_state8/1
  MATLAB Function7/4(y_voltage_per_switching_state) -> y_voltage_per_switching_state8/1
  MATLAB Function8/1(d_voltage_per_switching_state) -> d_voltage_per_switching_state7/1
  MATLAB Function8/2(q_voltage_per_switching_state) -> q_voltage_per_switching_state7/1
  MATLAB Function8/3(x_voltage_per_switching_state) -> x_voltage_per_switching_state7/1
  MATLAB Function8/4(y_voltage_per_switching_state) -> y_voltage_per_switching_state7/1
  MATLAB Function9/1(d_voltage_per_switching_state) -> d_voltage_per_switching_state6/1
  MATLAB Function9/2(q_voltage_per_switching_state) -> q_voltage_per_switching_state6/1
  MATLAB Function9/3(x_voltage_per_switching_state) -> x_voltage_per_switching_state6/1
  MATLAB Function9/4(y_voltage_per_switching_state) -> y_voltage_per_switching_state6/1
  Sincos_out1_buff/1 -> MATLAB Function9/1(sin_theta_el), MATLAB Function8/1(sin_theta_el), MATLAB Function7/1(sin_theta_el), MATLAB Function6/1(sin_theta_el), MATLAB Function5/1(sin_theta_el), MATLAB Function4/1(sin_theta_el), MATLAB Function3/1(sin_theta_el), MATLAB Function2/1(sin_theta_el), MATLAB Function15/1(sin_theta_el), MATLAB Function14/1(sin_theta_el), MATLAB Function13/1(sin_theta_el), MATLAB Function12/1(sin_theta_el), MATLAB Function11/1(sin_theta_el), MATLAB Function10/1(sin_theta_el), MATLAB Function1/1(sin_theta_el), MATLAB Function/1(sin_theta_el)
  Sincos_out2_buff/1 -> MATLAB Function9/2(cos_theta_el), MATLAB Function8/2(cos_theta_el), MATLAB Function7/2(cos_theta_el), MATLAB Function6/2(cos_theta_el), MATLAB Function5/2(cos_theta_el), MATLAB Function4/2(cos_theta_el), MATLAB Function3/2(cos_theta_el), MATLAB Function2/2(cos_theta_el), MATLAB Function15/2(cos_theta_el), MATLAB Function14/2(cos_theta_el), MATLAB Function13/2(cos_theta_el), MATLAB Function12/2(cos_theta_el), MATLAB Function11/2(cos_theta_el), MATLAB Function10/2(cos_theta_el), MATLAB Function1/2(cos_theta_el), MATLAB Function/2(cos_theta_el)
  Sincos/1(Out1) -> Sincos_out1_buff/1
  Sincos/2(Out2) -> Sincos_out2_buff/1
  theta_el_with_offset15/1 -> Sincos/1(In1)
  u_dc_link_voltage15/1 -> MATLAB Function9/3(u_dc_link_voltage), MATLAB Function8/3(u_dc_link_voltage), MATLAB Function7/3(u_dc_link_voltage), MATLAB Function6/3(u_dc_link_voltage), MATLAB Function5/3(u_dc_link_voltage), MATLAB Function4/3(u_dc_link_voltage), MATLAB Function3/3(u_dc_link_voltage), MATLAB Function2/3(u_dc_link_voltage), MATLAB Function15/3(u_dc_link_voltage), MATLAB Function14/3(u_dc_link_voltage), MATLAB Function13/3(u_dc_link_voltage), MATLAB Function12/3(u_dc_link_voltage), MATLAB Function11/3(u_dc_link_voltage), MATLAB Function10/3(u_dc_link_voltage), MATLAB Function1/3(u_dc_link_voltage), MATLAB Function/3(u_dc_link_voltage)
  Index 15/1 -> MATLAB Function9/4(Index), MATLAB Function8/4(Index), MATLAB Function7/4(Index), MATLAB Function6/4(Index), MATLAB Function5/4(Index), MATLAB Function4/4(Index), MATLAB Function3/4(Index), MATLAB Function2/4(Index), MATLAB Function15/4(Index), MATLAB Function14/4(Index), MATLAB Function13/4(Index), MATLAB Function12/4(Index), MATLAB Function11/4(Index), MATLAB Function10/4(Index), MATLAB Function1/4(Index), MATLAB Function/4(Index)

== system gm_parallel_phase_voltages_per_switching_state_6/Phase_voltages_per_switching_state/Detect Rise Positive/Positive ==
  u : Inport  OutDataTypeStr=boolean  SampleTime=1e-08
  Compare : RelationalOperator  Operator=>  OutDataTypeStr=boolean  ZeroCross=off
  Constant : Constant  DisableCoverage=on  Value=0  OutDataTypeStr=Inherit: Inherit via back propagation  SampleTime=-1  PreserveConstantTs=on
  y : Outport  SampleTime=1e-08
  wires:
  Compare/1 -> y/1
  Constant/1 -> Compare/2
  u/1 -> Compare/1

== system gm_parallel_phase_voltages_per_switching_state_6/Phase_voltages_per_switching_state/Detect Rise Positive1/Positive ==
  u : Inport  OutDataTypeStr=boolean  SampleTime=1e-08
  Compare : RelationalOperator  Operator=>  OutDataTypeStr=boolean  ZeroCross=off
  Constant : Constant  DisableCoverage=on  Value=0  OutDataTypeStr=Inherit: Inherit via back propagation  SampleTime=-1  PreserveConstantTs=on
  y : Outport  SampleTime=1e-08
  wires:
  Compare/1 -> y/1
  Constant/1 -> Compare/2
  u/1 -> Compare/1

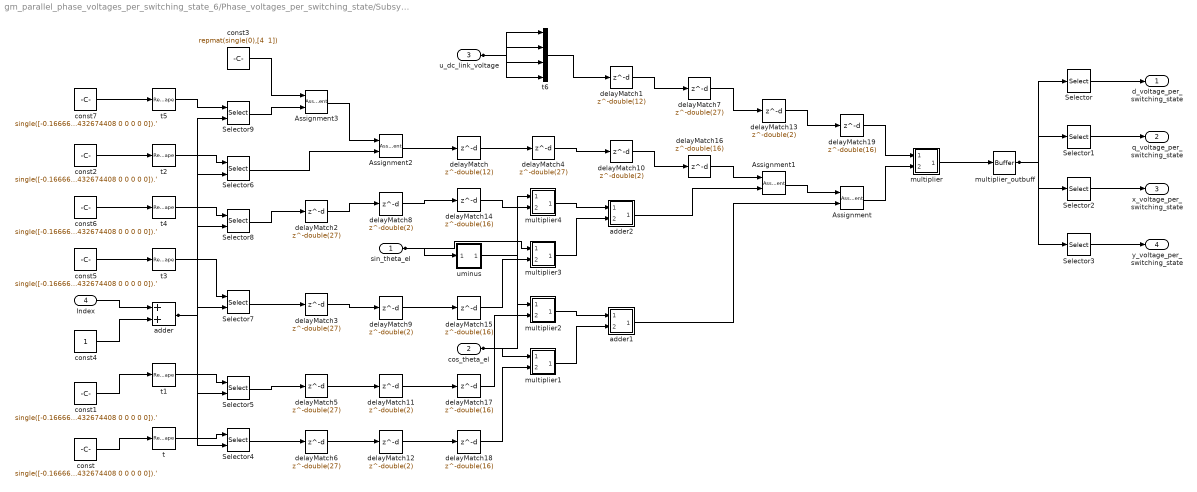
== system gm_parallel_phase_voltages_per_switching_state_6/Phase_voltages_per_switching_state/Subsystem/MATLAB Function ==
  sin_theta_el : Inport  OutDataTypeStr=single  PortDimensions=1  SampleTime=1e-08
  cos_theta_el : Inport  Port=2  OutDataTypeStr=single  PortDimensions=1  SampleTime=1e-08
  u_dc_link_voltage : Inport  Port=3  OutDataTypeStr=single  PortDimensions=1  SampleTime=1e-08
  Index : Inport  Port=4  OutDataTypeStr=int32  PortDimensions=1  SampleTime=1e-08
  Assignment : Assignment  NumberOfDimensions=2  SampleTime=1e-08  IndexOptions=Index vector (dialog),Index vector (dialog)  Indices=double(2),double(1)  OutputSizes=double(0),double(0)
  Assignment1 : Assignment  NumberOfDimensions=2  SampleTime=1e-08  IndexOptions=Index vector (dialog),Index vector (dialog)  Indices=double(1),double(1)  OutputSizes=double(0),double(0)
  Assignment2 : Assignment  NumberOfDimensions=2  SampleTime=1e-08  IndexOptions=Index vector (dialog),Index vector (dialog)  Indices=double(4),double(1)  OutputSizes=double(0),double(0)
  Assignment3 : Assignment  NumberOfDimensions=2  SampleTime=1e-08  IndexOptions=Index vector (dialog),Index vector (dialog)  Indices=double(3),double(1)  OutputSizes=double(0),double(0)
  Selector : Selector  NumberOfDimensions=2  SampleTime=1e-08  IndexOptions=Index vector (dialog),Index vector (dialog)  Indices=double(1),double(1)  OutputSizes=double(0),double(0)
  Selector1 : Selector  NumberOfDimensions=2  SampleTime=1e-08  IndexOptions=Index vector (dialog),Index vector (dialog)  Indices=double(2),double(1)  OutputSizes=double(0),double(0)
  Selector2 : Selector  NumberOfDimensions=2  SampleTime=1e-08  IndexOptions=Index vector (dialog),Index vector (dialog)  Indices=double(3),double(1)  OutputSizes=double(0),double(0)
  Selector3 : Selector  NumberOfDimensions=2  SampleTime=1e-08  IndexOptions=Index vector (dialog),Index vector (dialog)  Indices=double(4),double(1)  OutputSizes=double(0),double(0)
  Selector4 : Selector  NumberOfDimensions=2  SampleTime=1e-08  IndexOptions=Index vector (dialog),Index vector (port)  Indices=double(2),double(-1)  OutputSizes=double(0),double(0)
  Selector5 : Selector  NumberOfDimensions=2  SampleTime=1e-08  IndexOptions=Index vector (dialog),Index vector (port)  Indices=double(1),double(-1)  OutputSizes=double(0),double(0)
  Selector6 : Selector  NumberOfDimensions=2  SampleTime=1e-08  IndexOptions=Index vector (dialog),Index vector (port)  Indices=double(4),double(-1)  OutputSizes=double(0),double(0)
  Selector7 : Selector  NumberOfDimensions=2  SampleTime=1e-08  IndexOptions=Index vector (dialog),Index vector (port)  Indices=double(2),double(-1)  OutputSizes=double(0),double(0)
  Selector8 : Selector  NumberOfDimensions=2  SampleTime=1e-08  IndexOptions=Index vector (dialog),Index vector (port)  Indices=double(1),double(-1)  OutputSizes=double(0),double(0)
  Selector9 : Selector  NumberOfDimensions=2  SampleTime=1e-08  IndexOptions=Index vector (dialog),Index vector (port)  Indices=double(3),double(-1)  OutputSizes=double(0),double(0)
  adder : Sum  AccumDataTypeStr=int32  OutDataTypeStr=int32  RndMeth=Nearest  SaturateOnIntegerOverflow=on  SampleTime=1e-08
  adder1 : Subsystem
      mask Display: disp('NFP\nadd');
  adder2 : Subsystem
      mask Display: disp('NFP\nadd');
  const{,1..2,5..7} (6 alike) : Constant  Value=single([-0.1666666716337204 -0.28867512941360474 -0.1666666716337204 0.28867512941360474 0.1666666716337204 -0.28867512941360474 0.1666666716337204 0.28867512941360474 -0.3333333432674408 0 -0.3333333432674408 0 0 0 0 0]).'  VectorParams1D=off  OutDataTypeStr=single  SampleTime=1e-08
  const3 : Constant  Value="repmat(single(0),[4  1])"  VectorParams1D=off  OutDataTypeStr=single  SampleTime=1e-08
  const4 : Constant  VectorParams1D=off  OutDataTypeStr=int32  SampleTime=1e-08
  delayMatch : Delay  DelayLength=double(12)  InitialCondition=0  SampleTime=1e-08
  delayMatch1 : Delay  DelayLength=double(12)  InitialCondition=0  SampleTime=1e-08
  delayMatch{8..13} (6 alike) : Delay  DelayLength=double(2)  InitialCondition=0  SampleTime=1e-08
  delayMatch{14..19} (6 alike) : Delay  DelayLength=double(16)  InitialCondition=0  SampleTime=1e-08
  delayMatch{2..7} (6 alike) : Delay  DelayLength=double(27)  InitialCondition=0  SampleTime=1e-08
  multiplier : Subsystem
      mask Display: disp('NFP\nmul');
  multiplier1 : Subsystem
      mask Display: disp('NFP\nmul');
  multiplier2 : Subsystem
      mask Display: disp('NFP\nmul');
  multiplier3 : Subsystem
      mask Display: disp('NFP\nmul');
  multiplier4 : Subsystem
      mask Display: disp('NFP\nmul');
  multiplier_outbuff : hdlmdlgenlib/Buffer
      settings: SourceProductBaseCode=SL
  t{,1..5} (6 alike) : Reshape  OutputDimensionality=Customize  OutputDimensions=[4,4]
  t6 : Mux
  uminus : Subsystem
      mask Display: disp('NFP\numinus');
  d_voltage_per_switching_state : Outport  SampleTime=1e-08  VectorParamsAs1DForOutWhenUnconnected=off
  q_voltage_per_switching_state : Outport  Port=2  SampleTime=1e-08
  x_voltage_per_switching_state : Outport  Port=3  SampleTime=1e-08
  y_voltage_per_switching_state : Outport  Port=4  SampleTime=1e-08
  wires:
  Selector/1 -> d_voltage_per_switching_state/1
  Selector1/1 -> q_voltage_per_switching_state/1
  Selector2/1 -> x_voltage_per_switching_state/1
  Selector3/1 -> y_voltage_per_switching_state/1
  multiplier_outbuff/1 -> Selector3/1, Selector2/1, Selector1/1, Selector/1
  Assignment/1 -> multiplier/2(In2)
  Assignment1/1 -> Assignment/1
  delayMatch16/1 -> Assignment1/1
  delayMatch18/1 -> multiplier1/2(In2)
  delayMatch17/1 -> multiplier2/2(In2)
  Selector6/1 -> Assignment2/2
  Assignment3/1 -> Assignment2/1
  adder/1 -> Selector9/2, Selector8/2, Selector7/2, Selector6/2, Selector5/2, Selector4/2
  t/1 -> Selector4/1
  t1/1 -> Selector5/1
  delayMatch15/1 -> multiplier3/2(In2)
  delayMatch14/1 -> multiplier4/2(In2)
  t2/1 -> Selector6/1
  Selector9/1 -> Assignment3/2
  const3/1 -> Assignment3/1
  const4/1 -> adder/2
  t3/1 -> Selector7/1
  t4/1 -> Selector8/1
  t5/1 -> Selector9/1
  const/1 -> t/1
  const1/1 -> t1/1
  const2/1 -> t2/1
  const5/1 -> t3/1
  const6/1 -> t4/1
  const7/1 -> t5/1
  delayMatch19/1 -> multiplier/1(In1)
  multiplier/1(Out1) -> multiplier_outbuff/1
  adder1/1(Out1) -> Assignment/2
  multiplier1/1(Out1) -> adder1/2(In2)
  multiplier2/1(Out1) -> adder1/1(In1)
  adder2/1(Out1) -> Assignment1/2
  uminus/1(Out1) -> multiplier2/1(In1)
  multiplier3/1(Out1) -> adder2/2(In2)
  multiplier4/1(Out1) -> adder2/1(In1)
  Assignment2/1 -> delayMatch/1
  t6/1 -> delayMatch1/1
  Selector8/1 -> delayMatch2/1
  Selector7/1 -> delayMatch3/1
  delayMatch/1 -> delayMatch4/1
  Selector5/1 -> delayMatch5/1
  Selector4/1 -> delayMatch6/1
  delayMatch1/1 -> delayMatch7/1
  delayMatch2/1 -> delayMatch8/1
  delayMatch3/1 -> delayMatch9/1
  delayMatch4/1 -> delayMatch10/1
  delayMatch5/1 -> delayMatch11/1
  delayMatch6/1 -> delayMatch12/1
  delayMatch7/1 -> delayMatch13/1
  delayMatch8/1 -> delayMatch14/1
  delayMatch9/1 -> delayMatch15/1
  delayMatch10/1 -> delayMatch16/1
  delayMatch11/1 -> delayMatch17/1
  delayMatch12/1 -> delayMatch18/1
  delayMatch13/1 -> delayMatch19/1
  sin_theta_el/1 -> multiplier3/1(In1), uminus/1(In1)
  cos_theta_el/1 -> multiplier4/1(In1), multiplier1/1(In1)
  u_dc_link_voltage/1 -> t6/4, t6/3, t6/2, t6/1
  Index/1 -> adder/1
